simulink model "mrac"  (R2019b)
settings: Solver=FixedStepAuto  StartTime=0.0  StopTime=10  FixedStep=0.001  RelTol=1e-3
settings Model: Creator=jgakl

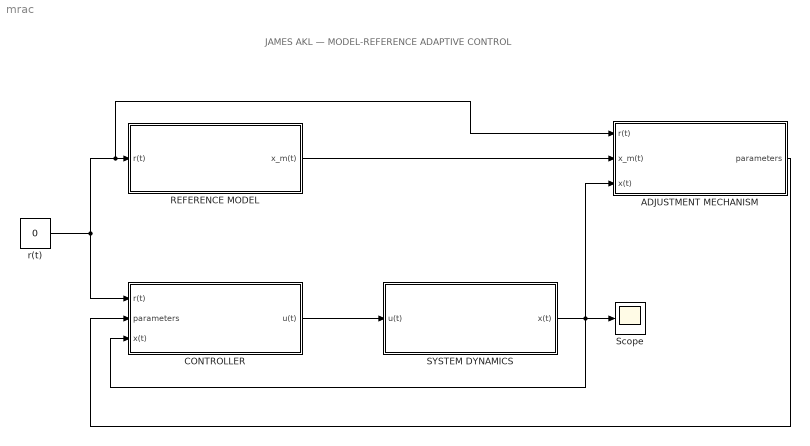
== system mrac ==
  note: JAMES AKL — MODEL-REFERENCE ADAPTIVE CONTROL
  ADJUSTMENT MECHANISM : Subsystem
  CONTROLLER : Subsystem
  REFERENCE MODEL : Subsystem
  SYSTEM DYNAMICS : Subsystem
  Scope : Scope
  r(t) : Constant  Value=0
  wires:
  SYSTEM DYNAMICS/1(x(t)) -> ADJUSTMENT MECHANISM/3(x(t)), CONTROLLER/3(x(t)), Scope/1
  CONTROLLER/1(u(t)) -> SYSTEM DYNAMICS/1(u(t))
  ADJUSTMENT MECHANISM/1(parameters) -> CONTROLLER/2(parameters)
  REFERENCE MODEL/1(x_m(t)) -> ADJUSTMENT MECHANISM/2(x_m(t))
  r(t)/1 -> CONTROLLER/1(r(t)), ADJUSTMENT MECHANISM/1(r(t)), REFERENCE MODEL/1(r(t))

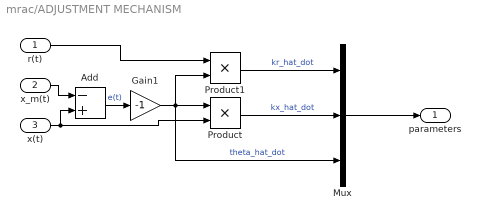
== system mrac/ADJUSTMENT MECHANISM ==
  r(t) : Inport
  x_m(t) : Inport  Port=2
  x(t) : Inport  Port=3
  Add : Sum  Inputs=-+
  Gain1 : Gain  Gain=-1
  Mux : Mux  Inputs=3
  Product : Product
  Product1 : Product
  parameters : Outport
  wires:
  x(t)/1 -> Product/2, Add/2
  x_m(t)/1 -> Add/1
  Add/1 -> Gain1/1  "e(t)"
  r(t)/1 -> Product1/1
  Product1/1 -> Mux/1  "kr_hat_dot"
  Product/1 -> Mux/2  "kx_hat_dot"
  Gain1/1 -> Mux/3, Product/1, Product1/2  "theta_hat_dot"
  Mux/1 -> parameters/1

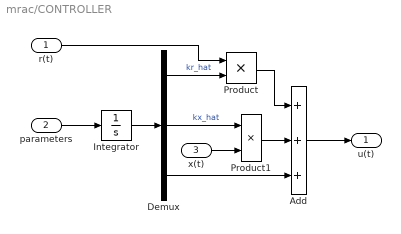
== system mrac/CONTROLLER ==
  r(t) : Inport
  parameters : Inport  Port=2
  x(t) : Inport  Port=3
  Add : Sum  Inputs=3
  Demux : Demux  Outputs=3
  Integrator : Integrator
  Product : Product
  Product1 : Product
  u(t) : Outport
  wires:
  parameters/1 -> Integrator/1
  Integrator/1 -> Demux/1
  Demux/1 -> Product/2  "kr_hat"
  r(t)/1 -> Product/1
  Demux/2 -> Product1/1  "kx_hat"
  x(t)/1 -> Product1/2
  Product/1 -> Add/1
  Product1/1 -> Add/2
  Demux/3 -> Add/3
  Add/1 -> u(t)/1

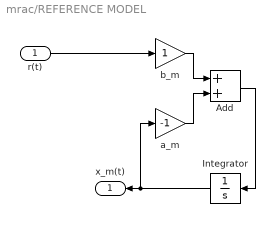
== system mrac/REFERENCE MODEL ==
  r(t) : Inport
  Add : Sum
  Integrator : Integrator  InitialCondition=-5
  a_m : Gain  Gain=-1
  b_m : Gain
  x_m(t) : Outport
  wires:
  r(t)/1 -> b_m/1
  a_m/1 -> Add/2
  b_m/1 -> Add/1
  Integrator/1 -> x_m(t)/1, a_m/1
  Add/1 -> Integrator/1

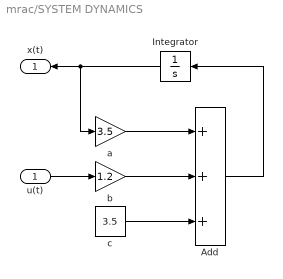
== system mrac/SYSTEM DYNAMICS ==
  u(t) : Inport
  Add : Sum  Inputs=+++
  Integrator : Integrator  InitialCondition=-5
  a : Gain  Gain=3.5
  b : Gain  Gain=1.2
  c : Constant  Value=3.5
  x(t) : Outport
  wires:
  c/1 -> Add/3
  b/1 -> Add/2
  a/1 -> Add/1
  u(t)/1 -> b/1
  Add/1 -> Integrator/1
  Integrator/1 -> a/1, x(t)/1
